simulink model "bai5"  (R2023a)
settings: Solver=VariableStepAuto  StartTime=0.0  StopTime=10  RelTol=1e-3
settings Model: Creator=Admin  LastModifiedBy=Admin

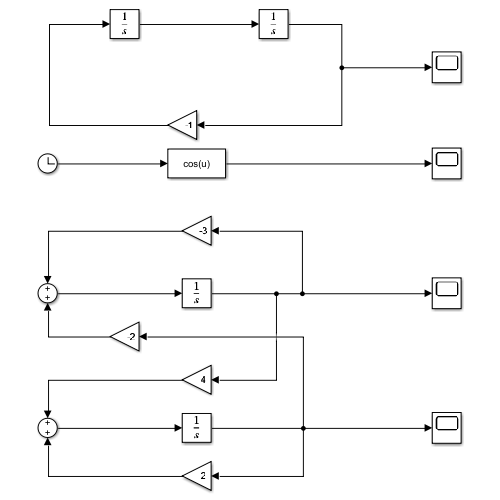
[thumbnail: Simulink's stored preview of the top-level diagram]
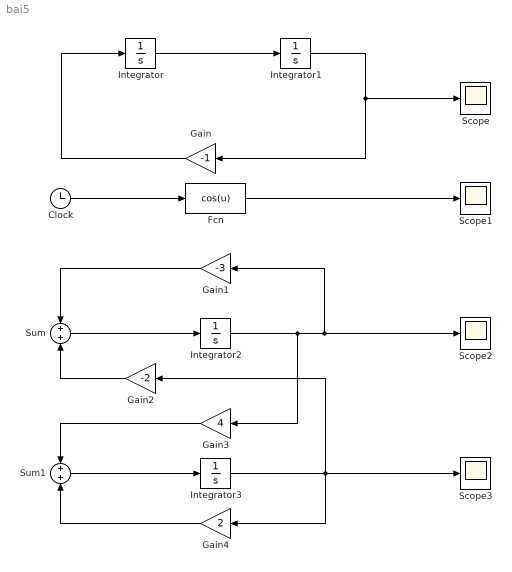
== system bai5 ==
  Clock : Clock
  Fcn : Fcn  Expr=cos(u)
  Gain : Gain  Gain=-1
  Gain1 : Gain  Gain=-3
  Gain2 : Gain  Gain=-2
  Gain3 : Gain  Gain=4
  Gain4 : Gain  Gain=2
  Integrator : Integrator
  Integrator1 : Integrator  InitialCondition=1
  Integrator2 : Integrator  InitialCondition=1
  Integrator3 : Integrator  InitialCondition=1
  Scope{,1..3} (4 alike) : Scope
  Sum : Sum  Inputs=+|+
  Sum1 : Sum  Inputs=+|+
  wires:
  Gain/1 -> Integrator/1
  Integrator/1 -> Integrator1/1
  Integrator1/1 -> Gain/1, Scope/1
  Clock/1 -> Fcn/1
  Fcn/1 -> Scope1/1
  Integrator3/1 -> Gain4/1, Scope3/1, Gain2/1
  Gain1/1 -> Sum/1
  Gain2/1 -> Sum/2
  Sum/1 -> Integrator2/1
  Sum1/1 -> Integrator3/1
  Gain3/1 -> Sum1/1
  Integrator2/1 -> Gain3/1, Gain1/1, Scope2/1
  Gain4/1 -> Sum1/2
